simulink library "XtremeDSPKit"  (Simulink 7.1)
libraries: xbsIndex_r4 x66, dspindex x2, dspmtrx3 x2
settings Model: Creator=shirazi  LastModifiedBy=sysgengroup

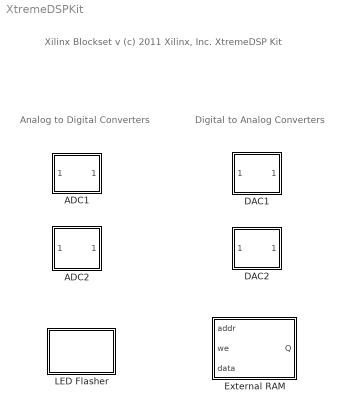
== system XtremeDSPKit ==
  note: Analog to Digital Converters
  note: Digital to Analog Converters
  note: Xilinx Blockset v
      | (c) 2011 Xilinx, Inc.
      |
      | XtremeDSP Kit
  ADC1 : Subsystem  mask(XtremeDSP Kit ADC1){period=1}
      mask prompts: period "Sample Period"
      mask help: Analog to Digital Converter #1
      mask init:
      | i = imread('xtreme.jpg');
      mask Help: eval('');xlDoc('-book','sysgen','-topic','XtremeDSP_Analog_to_Digital_Converter');
      mask Display: image(i)
  ADC2 : Subsystem  mask(XtremeDSP Kit  ADC2){period=1}
      mask prompts: period "Sample Period"
      mask help: Analog to Digital Converter #2
      mask init:
      | i = imread('xtreme.jpg');
      mask Help: eval('');xlDoc('-book','sysgen','-topic','XtremeDSP_Analog_to_Digital_Converter');
      mask Display: image(i)
  DAC1 : Subsystem  mask(XtremeDSP Kit DAC1){period=1}
      mask prompts: period "Sample Period"
      mask help: Digital to Analog Converter #1
      mask init:
      | i = imread('xtreme.jpg');
      mask Help: eval('');xlDoc('-book','sysgen','-topic','XtremeDSP_Digital_to_Analog_Converter');
      mask Display: image(i)
  DAC2 : Subsystem  mask(XtremeDSP Kit DAC2){period=1}
      mask prompts: period "Sample Period"
      mask help: Digital to Analog Converter #2
      mask init:
      | i = imread('xtreme.jpg');
      mask Help: eval('');xlDoc('-book','sysgen','-topic','XtremeDSP_Digital_to_Analog_Converter');
      mask Display: image(i)
  External RAM : Subsystem  mask(XtremeDSP Kit External Memory){zbt_data_read_arith_type=Unsigned, zbt_data_width=16, zbt_data_bin_pt=0}
      mask prompts: zbt_data_read_arith_type "Output Data Type"; zbt_data_width "Data Width"; zbt_data_bin_pt "Data Binary Point (from 0 to 16)"
      mask help: 256K x 16 External Memory
      mask init:
      | i = imread('xtreme.jpg');
      mask Help: eval('');xlDoc('-book','sysgen','-topic','XtremeDSP_External_RAM');
      mask StyleString: popup(Unsigned|Signed  (2's comp)),edit,edit
      mask Display:
      | image(i);
      | port_label ('input', 1, 'addr');
      | port_label ('input', 2, 'we');
      | port_label ('input', 3, 'data');
  LED Flasher : Subsystem  mask(LED Flasher){}
      mask help: This block will cause LEDs on the BenAdda to cycle through red, green, and yellow colors.
      mask init:
      | i = imread('LEDs.jpg');
      mask Help: eval('');xlDoc('-book','sysgen','-topic','XtremeDSP_LED_Flasher');
      mask Display: image(i)

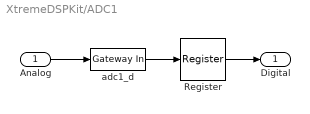
== system XtremeDSPKit/ADC1 ==
  Analog : Inport  OutDataType=sfix(16)  OutScaling=2^0
  Register : xbsIndex_r4/Register  init=0  rst=off  en=off  dbl_ovrd=off  block_type=register
      settings: xl_area=[0, 0, 0, 0, 0, 0, 0]  block_version=VER_STRING_GOES_HERE
  adc1_d : xbsIndex_r4/Gateway In  arith_type="Signed  (2's comp)"  n_bits=14  bin_pt=13  quantization="Round  (unbiased: +/- Inf)"  overflow=Saturate  period=period  dbl_ovrd=off  timing_constraint=None  locs_specified=off  LOCs={'w15', 'w14', 'w13', 'y15', 'y14', 'aa13', 'aa15', 'ab15', 'ac15', 'ad15', 'ac19', 'ac22', 'ad19', 'af20'}  block_type=gatewayin
      settings: infoedit="Gateway in block.  Converts inputs of type Simulink integer, double and fixed point to  Xilinx fixed point type.<P><P>Hardware notes:  In hardware these blocks become top level input ports."  xl_area=[0, 0, 0, 0, 0, 0, 0]  sginterface={'Nallatech'=>{'xdspkit'=>{'non_memory_mapped_port'=>'adc1_d'}},'Xilinx'=>{'jtaghwcosim'=>{'non_memory_mapped_port'=>'adc1_d'},'xdspkit'=>{'non_memory_mapped_port'=>'adc1_d'}}}  block_version=VER_STRING_GOES_HERE
  Digital : Outport  OutDataType=sfix(16)  OutScaling=2^0
  wires:
  Analog/1 -> adc1_d/1
  Register/1 -> Digital/1
  adc1_d/1 -> Register/1

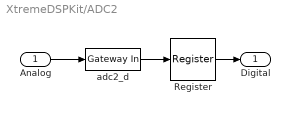
== system XtremeDSPKit/ADC2 ==
  Analog : Inport  OutDataType=sfix(16)  OutScaling=2^0
  Register : xbsIndex_r4/Register  init=0  rst=off  en=off  dbl_ovrd=off  block_type=register
      settings: xl_area=[0, 0, 0, 0, 0, 0, 0]  block_version=VER_STRING_GOES_HERE
  adc2_d : xbsIndex_r4/Gateway In  arith_type="Signed  (2's comp)"  n_bits=14  bin_pt=13  quantization="Round  (unbiased: +/- Inf)"  overflow=Saturate  period=period  dbl_ovrd=off  timing_constraint=None  locs_specified=off  LOCs={'w12', 'y10', 'y8', 'aa8', 'aa7', 'ab8', 'ab7', 'ab6', 'ac7', 'ac6', 'ac5', 'ad7', 'ad6', 'ad12'}  block_type=gatewayin
      settings: infoedit="Gateway in block.  Converts inputs of type Simulink integer, double and fixed point to  Xilinx fixed point type.<P><P>Hardware notes:  In hardware these blocks become top level input ports."  xl_area=[0, 0, 0, 0, 0, 0, 0]  sginterface={'Nallatech'=>{'xdspkit'=>{'non_memory_mapped_port'=>'adc2_d'}},'Xilinx'=>{'jtaghwcosim'=>{'non_memory_mapped_port'=>'adc2_d'},'xdspkit'=>{'non_memory_mapped_port'=>'adc2_d'}}}  block_version=VER_STRING_GOES_HERE
  Digital : Outport  OutDataType=sfix(16)  OutScaling=2^0
  wires:
  Analog/1 -> adc2_d/1
  Register/1 -> Digital/1
  adc2_d/1 -> Register/1

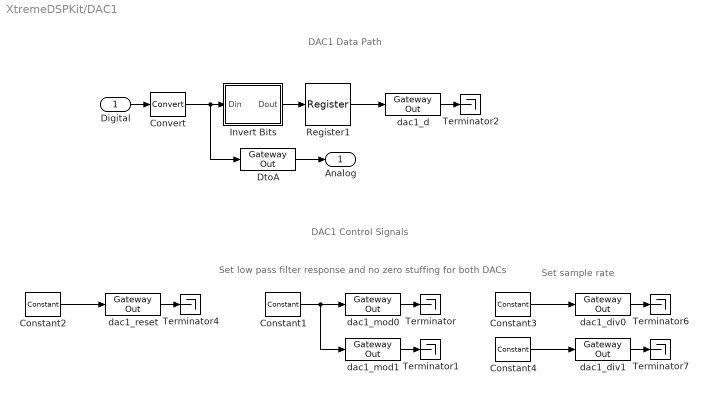
== system XtremeDSPKit/DAC1 ==
  note: DAC1 Data Path
  note: DAC1 Control Signals
  note: Set low pass filter response and
      | no zero stuffing for both DACs
  note: Set sample rate
  Digital : Inport  OutDataType=sfix(16)  OutScaling=2^0
  Constant1 : xbsIndex_r4/Constant  arith_type=Unsigned  const=0  n_bits=1  bin_pt=0  explicit_period=on  period=period  equ=P=C  opselect=C  inp2=PCIN>>17  opr=+  inp1=P  carry=CIN  dbl_ovrd=off  block_type=constant
      settings: block_version=VER_STRING_GOES_HERE
  Constant2 : xbsIndex_r4/Constant  arith_type=Unsigned  const=0  n_bits=1  bin_pt=0  explicit_period=on  period=period  equ=P=C  opselect=C  inp2=PCIN>>17  opr=+  inp1=P  carry=CIN  dbl_ovrd=off  block_type=constant
      settings: block_version=VER_STRING_GOES_HERE
  Constant3 : xbsIndex_r4/Constant  arith_type=Unsigned  const=1  n_bits=1  bin_pt=0  explicit_period=on  period=period  equ=P=C  opselect=C  inp2=PCIN>>17  opr=+  inp1=P  carry=CIN  dbl_ovrd=off  block_type=constant
      settings: block_version=VER_STRING_GOES_HERE
  Constant4 : xbsIndex_r4/Constant  arith_type=Unsigned  const=0  n_bits=1  bin_pt=0  explicit_period=on  period=period  equ=P=C  opselect=C  inp2=PCIN>>17  opr=+  inp1=P  carry=CIN  dbl_ovrd=off  block_type=constant
      settings: block_version=VER_STRING_GOES_HERE
  Convert : xbsIndex_r4/Convert  arith_type="Signed  (2's comp)"  n_bits=14  bin_pt=13  quantization=Truncate  overflow=Wrap  latency=0  dbl_ovrd=off  pipeline=off  block_type=convert
      settings: infoedit=The input is presented at the output after quantization and overflow effects.<P><P>Hardware notes: Additional hardware is used when rounding or saturation is selected and output width is less than the input width.  xl_area=[0, 0, 0, 0, 0, 0, 0]  block_version=VER_STRING_GOES_HERE
  DtoA : xbsIndex_r4/Gateway Out  hdl_port=off  timing_constraint=None  locs_specified=off  LOCs={}  block_type=gatewayout
      settings: infoedit="Gateway out block.  Converts Xilinx fixed point inputs into ouputs of type Simulink integer, double, or fixed point.<P><P>Hardware notes:  In hardware these blocks become top level output ports or are discarded, depending on how they are configured."  xl_area=[0, 0, 0, 0, 0, 0, 0]  block_version=VER_STRING_GOES_HERE
  Invert Bits : Subsystem
  Register1 : xbsIndex_r4/Register  init=0  rst=off  en=off  dbl_ovrd=off  block_type=register
      settings: xl_area=[0, 0, 0, 0, 0, 0, 0]  block_version=VER_STRING_GOES_HERE
  Terminator{,1..2,4,6..7} (6 alike) : Terminator
  dac1_d : xbsIndex_r4/Gateway Out  hdl_port=on  timing_constraint=None  locs_specified=off  LOCs={'p19', 'p20', 'p21', 'p22', 'p23', 'r19', 'r23', 'r24', 't19', 'u21', 'u22', 'u23', 'u24', 'v24'}  block_type=gatewayout
      settings: infoedit="Gateway out block.  Converts Xilinx fixed point inputs into ouputs of type Simulink integer, double, or fixed point.<P><P>Hardware notes:  In hardware these blocks become top level output ports or are discarded, depending on how they are configured."  xl_area=[0, 0, 0, 0, 0, 0, 0]  sginterface={'Nallatech'=>{'xdspkit'=>{'non_memory_mapped_port'=>'dac1_d'}},'Xilinx'=>{'jtaghwcosim'=>{'non_memory_mapped_port'=>'dac1_d'},'xdspkit'=>{'non_memory_mapped_port'=>'dac1_d'}}}  block_version=VER_STRING_GOES_HERE
  dac1_div0 : xbsIndex_r4/Gateway Out  hdl_port=on  timing_constraint=None  locs_specified=off  LOCs={'t20'}  block_type=gatewayout
      settings: infoedit="Gateway out block.  Converts Xilinx fixed point inputs into ouputs of type Simulink integer, double, or fixed point.<P><P>Hardware notes:  In hardware these blocks become top level output ports or are discarded, depending on how they are configured."  xl_area=[0, 0, 0, 0, 0, 0, 0]  sginterface={'Nallatech'=>{'xdspkit'=>{'non_memory_mapped_port'=>'dac1_div0'}},'Xilinx'=>{'jtaghwcosim'=>{'non_memory_mapped_port'=>'dac1_div0'},'xdspkit'=>{'non_memory_mapped_port'=>'dac1_div0'}}}  block_version=VER_STRING_GOES_HERE
  dac1_div1 : xbsIndex_r4/Gateway Out  hdl_port=on  timing_constraint=None  locs_specified=off  LOCs={'t24'}  block_type=gatewayout
      settings: infoedit="Gateway out block.  Converts Xilinx fixed point inputs into ouputs of type Simulink integer, double, or fixed point.<P><P>Hardware notes:  In hardware these blocks become top level output ports or are discarded, depending on how they are configured."  xl_area=[0, 0, 0, 0, 0, 0, 0]  sginterface={'Nallatech'=>{'xdspkit'=>{'non_memory_mapped_port'=>'dac1_div1'}},'Xilinx'=>{'jtaghwcosim'=>{'non_memory_mapped_port'=>'dac1_div1'},'xdspkit'=>{'non_memory_mapped_port'=>'dac1_div1'}}}  block_version=VER_STRING_GOES_HERE
  dac1_mod0 : xbsIndex_r4/Gateway Out  hdl_port=on  timing_constraint=None  locs_specified=off  LOCs={'r21'}  block_type=gatewayout
      settings: infoedit="Gateway out block.  Converts Xilinx fixed point inputs into ouputs of type Simulink integer, double, or fixed point.<P><P>Hardware notes:  In hardware these blocks become top level output ports or are discarded, depending on how they are configured."  xl_area=[0, 0, 0, 0, 0, 0, 0]  sginterface={'Nallatech'=>{'xdspkit'=>{'non_memory_mapped_port'=>'dac1_mod0'}},'Xilinx'=>{'jtaghwcosim'=>{'non_memory_mapped_port'=>'dac1_mod0'},'xdspkit'=>{'non_memory_mapped_port'=>'dac1_mod0'}}}  block_version=VER_STRING_GOES_HERE
  dac1_mod1 : xbsIndex_r4/Gateway Out  hdl_port=on  timing_constraint=None  locs_specified=off  LOCs={'r22'}  block_type=gatewayout
      settings: infoedit="Gateway out block.  Converts Xilinx fixed point inputs into ouputs of type Simulink integer, double, or fixed point.<P><P>Hardware notes:  In hardware these blocks become top level output ports or are discarded, depending on how they are configured."  xl_area=[0, 0, 0, 0, 0, 0, 0]  sginterface={'Nallatech'=>{'xdspkit'=>{'non_memory_mapped_port'=>'dac1_mod1'}},'Xilinx'=>{'jtaghwcosim'=>{'non_memory_mapped_port'=>'dac1_mod1'},'xdspkit'=>{'non_memory_mapped_port'=>'dac1_mod1'}}}  block_version=VER_STRING_GOES_HERE
  dac1_reset : xbsIndex_r4/Gateway Out  hdl_port=on  timing_constraint=None  locs_specified=off  LOCs={'v23'}  block_type=gatewayout
      settings: infoedit="Gateway out block.  Converts Xilinx fixed point inputs into ouputs of type Simulink integer, double, or fixed point.<P><P>Hardware notes:  In hardware these blocks become top level output ports or are discarded, depending on how they are configured."  xl_area=[0, 0, 0, 0, 0, 0, 0]  sginterface={'Nallatech'=>{'xdspkit'=>{'non_memory_mapped_port'=>'dac1_reset'}},'Xilinx'=>{'jtaghwcosim'=>{'non_memory_mapped_port'=>'dac1_reset'},'xdspkit'=>{'non_memory_mapped_port'=>'dac1_reset'}}}  block_version=VER_STRING_GOES_HERE
  Analog : Outport  OutDataType=sfix(16)  OutScaling=2^0
  wires:
  DtoA/1 -> Analog/1
  dac1_d/1 -> Terminator2/1
  Constant4/1 -> dac1_div1/1
  dac1_div1/1 -> Terminator7/1
  dac1_div0/1 -> Terminator6/1
  Constant3/1 -> dac1_div0/1
  dac1_reset/1 -> Terminator4/1
  Constant2/1 -> dac1_reset/1
  dac1_mod1/1 -> Terminator1/1
  dac1_mod0/1 -> Terminator/1
  Constant1/1 -> dac1_mod1/1, dac1_mod0/1
  Digital/1 -> Convert/1
  Register1/1 -> dac1_d/1
  Invert Bits/1(Dout) -> Register1/1
  Convert/1 -> DtoA/1, Invert Bits/1(Din)

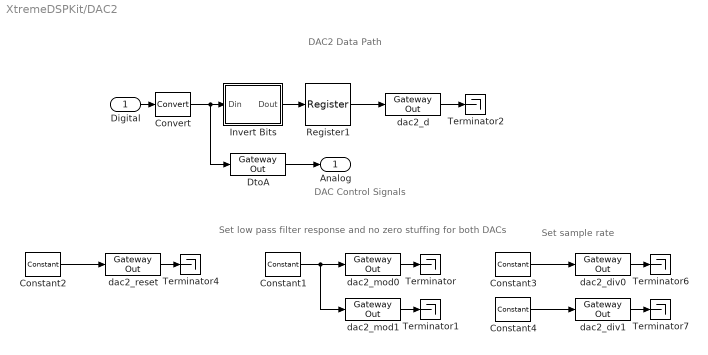
== system XtremeDSPKit/DAC2 ==
  note: Set sample rate
  note: Set low pass filter response and
      | no zero stuffing for both DACs
  note: DAC Control Signals
  note: DAC2 Data Path
  Digital : Inport  OutDataType=sfix(16)  OutScaling=2^0
  Constant1 : xbsIndex_r4/Constant  arith_type=Unsigned  const=0  n_bits=1  bin_pt=0  explicit_period=on  period=period  equ=P=C  opselect=C  inp2=PCIN>>17  opr=+  inp1=P  carry=CIN  dbl_ovrd=off  block_type=constant
      settings: block_version=VER_STRING_GOES_HERE
  Constant2 : xbsIndex_r4/Constant  arith_type=Unsigned  const=0  n_bits=1  bin_pt=0  explicit_period=on  period=period  equ=P=C  opselect=C  inp2=PCIN>>17  opr=+  inp1=P  carry=CIN  dbl_ovrd=off  block_type=constant
      settings: block_version=VER_STRING_GOES_HERE
  Constant3 : xbsIndex_r4/Constant  arith_type=Unsigned  const=1  n_bits=1  bin_pt=0  explicit_period=on  period=period  equ=P=C  opselect=C  inp2=PCIN>>17  opr=+  inp1=P  carry=CIN  dbl_ovrd=off  block_type=constant
      settings: block_version=VER_STRING_GOES_HERE
  Constant4 : xbsIndex_r4/Constant  arith_type=Unsigned  const=0  n_bits=1  bin_pt=0  explicit_period=on  period=period  equ=P=C  opselect=C  inp2=PCIN>>17  opr=+  inp1=P  carry=CIN  dbl_ovrd=off  block_type=constant
      settings: block_version=VER_STRING_GOES_HERE
  Convert : xbsIndex_r4/Convert  arith_type="Signed  (2's comp)"  n_bits=14  bin_pt=13  quantization=Truncate  overflow=Wrap  latency=0  dbl_ovrd=off  pipeline=off  block_type=convert
      settings: infoedit=The input is presented at the output after quantization and overflow effects.<P><P>Hardware notes: Additional hardware is used when rounding or saturation is selected and output width is less than the input width.  xl_area=[0, 0, 0, 0, 0, 0, 0]  block_version=VER_STRING_GOES_HERE
  DtoA : xbsIndex_r4/Gateway Out  hdl_port=off  timing_constraint=None  locs_specified=off  LOCs={}  block_type=gatewayout
      settings: infoedit="Gateway out block.  Converts Xilinx fixed point inputs into ouputs of type Simulink integer, double, or fixed point.<P><P>Hardware notes:  In hardware these blocks become top level output ports or are discarded, depending on how they are configured."  xl_area=[0, 0, 0, 0, 0, 0, 0]  block_version=VER_STRING_GOES_HERE
  Invert Bits : Subsystem
  Register1 : xbsIndex_r4/Register  init=0  rst=off  en=off  dbl_ovrd=off  block_type=register
      settings: xl_area=[0, 0, 0, 0, 0, 0, 0]  block_version=VER_STRING_GOES_HERE
  Terminator{,1..2,4,6..7} (6 alike) : Terminator
  dac2_d : xbsIndex_r4/Gateway Out  hdl_port=on  timing_constraint=None  locs_specified=off  LOCs={'y19', 'y20', 'y22', 'aa19', 'aa20', 'aa22', 'aa23', 'aa24', 'ab19', 'ab20', 'ab23', 'ab24', 'ac21', 'ad21'}  block_type=gatewayout
      settings: infoedit="Gateway out block.  Converts Xilinx fixed point inputs into ouputs of type Simulink integer, double, or fixed point.<P><P>Hardware notes:  In hardware these blocks become top level output ports or are discarded, depending on how they are configured."  xl_area=[0, 0, 0, 0, 0, 0, 0]  sginterface={'Nallatech'=>{'xdspkit'=>{'non_memory_mapped_port'=>'dac2_d'}},'Xilinx'=>{'jtaghwcosim'=>{'non_memory_mapped_port'=>'dac2_d'},'xdspkit'=>{'non_memory_mapped_port'=>'dac2_d'}}}  block_version=VER_STRING_GOES_HERE
  dac2_div0 : xbsIndex_r4/Gateway Out  hdl_port=on  timing_constraint=None  locs_specified=off  LOCs={'ac17'}  block_type=gatewayout
      settings: infoedit="Gateway out block.  Converts Xilinx fixed point inputs into ouputs of type Simulink integer, double, or fixed point.<P><P>Hardware notes:  In hardware these blocks become top level output ports or are discarded, depending on how they are configured."  xl_area=[0, 0, 0, 0, 0, 0, 0]  sginterface={'Nallatech'=>{'xdspkit'=>{'non_memory_mapped_port'=>'dac2_div0'}},'Xilinx'=>{'jtaghwcosim'=>{'non_memory_mapped_port'=>'dac2_div0'},'xdspkit'=>{'non_memory_mapped_port'=>'dac2_div0'}}}  block_version=VER_STRING_GOES_HERE
  dac2_div1 : xbsIndex_r4/Gateway Out  hdl_port=on  timing_constraint=None  locs_specified=off  LOCs={'ad17'}  block_type=gatewayout
      settings: infoedit="Gateway out block.  Converts Xilinx fixed point inputs into ouputs of type Simulink integer, double, or fixed point.<P><P>Hardware notes:  In hardware these blocks become top level output ports or are discarded, depending on how they are configured."  xl_area=[0, 0, 0, 0, 0, 0, 0]  sginterface={'Nallatech'=>{'xdspkit'=>{'non_memory_mapped_port'=>'dac2_div1'}},'Xilinx'=>{'jtaghwcosim'=>{'non_memory_mapped_port'=>'dac2_div1'},'xdspkit'=>{'non_memory_mapped_port'=>'dac2_div1'}}}  block_version=VER_STRING_GOES_HERE
  dac2_mod0 : xbsIndex_r4/Gateway Out  hdl_port=on  timing_constraint=None  locs_specified=off  LOCs={'t22'}  block_type=gatewayout
      settings: infoedit="Gateway out block.  Converts Xilinx fixed point inputs into ouputs of type Simulink integer, double, or fixed point.<P><P>Hardware notes:  In hardware these blocks become top level output ports or are discarded, depending on how they are configured."  xl_area=[0, 0, 0, 0, 0, 0, 0]  sginterface={'Nallatech'=>{'xdspkit'=>{'non_memory_mapped_port'=>'dac2_mod0'}},'Xilinx'=>{'jtaghwcosim'=>{'non_memory_mapped_port'=>'dac2_mod0'},'xdspkit'=>{'non_memory_mapped_port'=>'dac2_mod0'}}}  block_version=VER_STRING_GOES_HERE
  dac2_mod1 : xbsIndex_r4/Gateway Out  hdl_port=on  timing_constraint=None  locs_specified=off  LOCs={'t21'}  block_type=gatewayout
      settings: infoedit="Gateway out block.  Converts Xilinx fixed point inputs into ouputs of type Simulink integer, double, or fixed point.<P><P>Hardware notes:  In hardware these blocks become top level output ports or are discarded, depending on how they are configured."  xl_area=[0, 0, 0, 0, 0, 0, 0]  sginterface={'Nallatech'=>{'xdspkit'=>{'non_memory_mapped_port'=>'dac2_mod1'}},'Xilinx'=>{'jtaghwcosim'=>{'non_memory_mapped_port'=>'dac2_mod1'},'xdspkit'=>{'non_memory_mapped_port'=>'dac2_mod1'}}}  block_version=VER_STRING_GOES_HERE
  dac2_reset : xbsIndex_r4/Gateway Out  hdl_port=on  timing_constraint=None  locs_specified=off  LOCs={'u20'}  block_type=gatewayout
      settings: infoedit="Gateway out block.  Converts Xilinx fixed point inputs into ouputs of type Simulink integer, double, or fixed point.<P><P>Hardware notes:  In hardware these blocks become top level output ports or are discarded, depending on how they are configured."  xl_area=[0, 0, 0, 0, 0, 0, 0]  sginterface={'Nallatech'=>{'xdspkit'=>{'non_memory_mapped_port'=>'dac2_reset'}},'Xilinx'=>{'jtaghwcosim'=>{'non_memory_mapped_port'=>'dac2_reset'},'xdspkit'=>{'non_memory_mapped_port'=>'dac2_reset'}}}  block_version=VER_STRING_GOES_HERE
  Analog : Outport  OutDataType=sfix(16)  OutScaling=2^0
  wires:
  DtoA/1 -> Analog/1
  dac2_d/1 -> Terminator2/1
  Invert Bits/1(Dout) -> Register1/1
  Register1/1 -> dac2_d/1
  Digital/1 -> Convert/1
  Constant1/1 -> dac2_mod0/1, dac2_mod1/1
  dac2_mod0/1 -> Terminator/1
  dac2_mod1/1 -> Terminator1/1
  Constant2/1 -> dac2_reset/1
  dac2_reset/1 -> Terminator4/1
  Constant3/1 -> dac2_div0/1
  dac2_div0/1 -> Terminator6/1
  dac2_div1/1 -> Terminator7/1
  Constant4/1 -> dac2_div1/1
  Convert/1 -> DtoA/1, Invert Bits/1(Din)

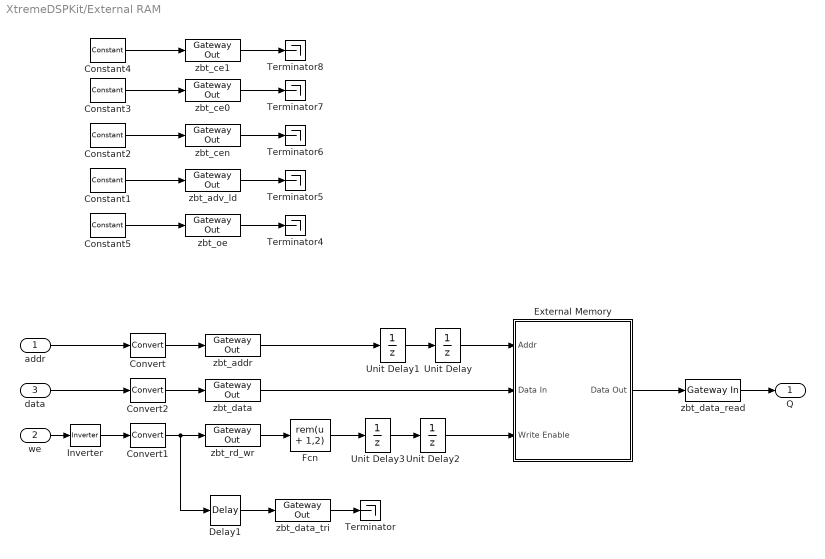
== system XtremeDSPKit/External RAM ==
  addr : Inport  OutDataType=sfix(16)  OutScaling=2^0
  we : Inport  Port=2  OutDataType=sfix(16)  OutScaling=2^0
  data : Inport  Port=3  OutDataType=sfix(16)  OutScaling=2^0
  Constant{1..5} (5 alike) : xbsIndex_r4/Constant  arith_type=Unsigned  const=0  n_bits=1  bin_pt=0  explicit_period=on  period=1  equ=P=C  opselect=C  inp2=PCIN>>17  opr=+  inp1=P  carry=CIN  dbl_ovrd=off  block_type=constant
      settings: block_version=VER_STRING_GOES_HERE
  Convert : xbsIndex_r4/Convert  arith_type=Unsigned  n_bits=18  bin_pt=0  quantization=Truncate  overflow=Wrap  latency=0  dbl_ovrd=off  pipeline=off  block_type=convert
      settings: infoedit=The input is presented at the output after quantization and overflow effects.<P><P>Hardware notes: Additional hardware is used when rounding or saturation is selected and output width is less than the input width.  xl_area=[0, 0, 0, 0, 0, 0, 0]  block_version=VER_STRING_GOES_HERE
  Convert1 : xbsIndex_r4/Convert  arith_type=Boolean  n_bits=1  bin_pt=0  quantization=Truncate  overflow=Wrap  latency=0  dbl_ovrd=off  pipeline=off  block_type=convert
      settings: infoedit=The input is presented at the output after quantization and overflow effects.<P><P>Hardware notes: Additional hardware is used when rounding or saturation is selected and output width is less than the input width.  xl_area=[0, 0, 0, 0, 0, 0, 0]  block_version=VER_STRING_GOES_HERE
  Convert2 : xbsIndex_r4/Convert  arith_type="Signed  (2's comp)"  n_bits=zbt_data_width  bin_pt=zbt_data_bin_pt  quantization=Truncate  overflow=Wrap  latency=0  dbl_ovrd=off  pipeline=off  block_type=convert
      settings: infoedit=The input is presented at the output after quantization and overflow effects.<P><P>Hardware notes: Additional hardware is used when rounding or saturation is selected and output width is less than the input width.  xl_area=[0, 0, 0, 0, 0, 0, 0]  block_version=VER_STRING_GOES_HERE
  Delay1 : xbsIndex_r4/Delay  en=off  latency=2  dbl_ovrd=off  reg_retiming=off  block_type=delay
      settings: infoedit="Delay line having  configurable length.<P><P>Hardware notes: A delay line is a chain, each link of which is an SRL16 followed by a flip-flop. If register retiming is enabled, the delay line is a chain of flip-flops."  xl_area=[0, 0, 0, 0, 0, 0, 0]  block_version=VER_STRING_GOES_HERE
  External Memory : Subsystem  mask{depth=4096, init_vec=0*(0:4095)}
      mask prompts: depth "Memory Depth"; init_vec "Initial Value"
  Fcn : Fcn  Expr=rem(u + 1,2)
  Inverter : xbsIndex_r4/Inverter  en=off  latency=0  dbl_ovrd=off  block_type=inv
      settings: xl_area=[0, 0, 0, 0, 0, 0, 0]  block_version=VER_STRING_GOES_HERE
  Terminator{,4..8} (6 alike) : Terminator
  Unit Delay{,1..3} (4 alike) : UnitDelay
  zbt_addr : xbsIndex_r4/Gateway Out  hdl_port=on  timing_constraint=None  locs_specified=off  LOCs={'A5','B9','A9','C1','A3','G6','E9','A6','A7','A8','B8','B1','B3','D9','B5','B4','B6','C2'}  block_type=gatewayout
      settings: infoedit="Gateway out block.  Converts Xilinx fixed point inputs into ouputs of type Simulink integer, double, or fixed point.<P><P>Hardware notes:  In hardware these blocks become top level output ports or are discarded, depending on how they are configured."  xl_area=[0, 0, 0, 0, 0, 0, 0]  sginterface={'Nallatech'=>{'xdspkit'=>{'non_memory_mapped_port'=>'zbt_addr'}},'Xilinx'=>{'jtaghwcosim'=>{'non_memory_mapped_port'=>'zbt_addr'},'xdspkit'=>{'non_memory_mapped_port'=>'zbt_addr'}}}  block_version=VER_STRING_GOES_HERE
  zbt_adv_ld : xbsIndex_r4/Gateway Out  hdl_port=on  timing_constraint=None  locs_specified=off  LOCs={'B15'}  block_type=gatewayout
      settings: infoedit="Gateway out block.  Converts Xilinx fixed point inputs into ouputs of type Simulink integer, double, or fixed point.<P><P>Hardware notes:  In hardware these blocks become top level output ports or are discarded, depending on how they are configured."  xl_area=[0, 0, 0, 0, 0, 0, 0]  sginterface={'Nallatech'=>{'xdspkit'=>{'non_memory_mapped_port'=>'zbt_adv_ld'}},'Xilinx'=>{'jtaghwcosim'=>{'non_memory_mapped_port'=>'zbt_adv_ld'},'xdspkit'=>{'non_memory_mapped_port'=>'zbt_adv_ld'}}}  block_version=VER_STRING_GOES_HERE
  zbt_ce0 : xbsIndex_r4/Gateway Out  hdl_port=on  timing_constraint=None  locs_specified=off  LOCs={'A18'}  block_type=gatewayout
      settings: infoedit="Gateway out block.  Converts Xilinx fixed point inputs into ouputs of type Simulink integer, double, or fixed point.<P><P>Hardware notes:  In hardware these blocks become top level output ports or are discarded, depending on how they are configured."  xl_area=[0, 0, 0, 0, 0, 0, 0]  sginterface={'Nallatech'=>{'xdspkit'=>{'non_memory_mapped_port'=>'zbt_ce0'}},'Xilinx'=>{'jtaghwcosim'=>{'non_memory_mapped_port'=>'zbt_ce0'},'xdspkit'=>{'non_memory_mapped_port'=>'zbt_ce0'}}}  block_version=VER_STRING_GOES_HERE
  zbt_ce1 : xbsIndex_r4/Gateway Out  hdl_port=on  timing_constraint=None  locs_specified=off  LOCs={'A19'}  block_type=gatewayout
      settings: infoedit="Gateway out block.  Converts Xilinx fixed point inputs into ouputs of type Simulink integer, double, or fixed point.<P><P>Hardware notes:  In hardware these blocks become top level output ports or are discarded, depending on how they are configured."  xl_area=[0, 0, 0, 0, 0, 0, 0]  sginterface={'Nallatech'=>{'xdspkit'=>{'non_memory_mapped_port'=>'zbt_ce1'}},'Xilinx'=>{'jtaghwcosim'=>{'non_memory_mapped_port'=>'zbt_ce1'},'xdspkit'=>{'non_memory_mapped_port'=>'zbt_ce1'}}}  block_version=VER_STRING_GOES_HERE
  zbt_cen : xbsIndex_r4/Gateway Out  hdl_port=on  timing_constraint=None  locs_specified=off  LOCs={'C15'}  block_type=gatewayout
      settings: infoedit="Gateway out block.  Converts Xilinx fixed point inputs into ouputs of type Simulink integer, double, or fixed point.<P><P>Hardware notes:  In hardware these blocks become top level output ports or are discarded, depending on how they are configured."  xl_area=[0, 0, 0, 0, 0, 0, 0]  sginterface={'Nallatech'=>{'xdspkit'=>{'non_memory_mapped_port'=>'zbt_cen'}},'Xilinx'=>{'jtaghwcosim'=>{'non_memory_mapped_port'=>'zbt_cen'},'xdspkit'=>{'non_memory_mapped_port'=>'zbt_cen'}}}  block_version=VER_STRING_GOES_HERE
  zbt_data : xbsIndex_r4/Gateway Out  hdl_port=on  timing_constraint=None  locs_specified=off  LOCs={'B21','B22','A22','B23','B19','C19','A20','A21','A23','B24','A24','A25','E18','D18','C18','B18'}  block_type=gatewayout
      settings: infoedit="Gateway out block.  Converts Xilinx fixed point inputs into ouputs of type Simulink integer, double, or fixed point.<P><P>Hardware notes:  In hardware these blocks become top level output ports or are discarded, depending on how they are configured."  xl_area=[0, 0, 0, 0, 0, 0, 0]  sginterface={'Nallatech'=>{'xdspkit'=>{'non_memory_mapped_port'=>'zbt_data'}},'Xilinx'=>{'jtaghwcosim'=>{'non_memory_mapped_port'=>'zbt_data'},'xdspkit'=>{'non_memory_mapped_port'=>'zbt_data'}}}  block_version=VER_STRING_GOES_HERE
  zbt_data_read : xbsIndex_r4/Gateway In  arith_type_sgadvanced=zbt_data_read_arith_type  arith_type=Unsigned  n_bits=zbt_data_width  bin_pt=zbt_data_bin_pt  quantization="Round  (unbiased: +/- Inf)"  overflow=Saturate  period=1  dbl_ovrd=off  timing_constraint=None  locs_specified=off  LOCs={}  block_type=gatewayin
      settings: infoedit="Gateway in block.  Converts inputs of type Simulink integer, double and fixed point to  Xilinx fixed point type.<P><P>Hardware notes:  In hardware these blocks become top level input ports."  xl_area=[0, 0, 0, 0, 0, 0, 0]  sginterface={'Nallatech'=>{'xdspkit'=>{'non_memory_mapped_port'=>'zbt_data_read'}},'Xilinx'=>{'jtaghwcosim'=>{'non_memory_mapped_port'=>'zbt_data_read'},'xdspkit'=>{'non_memory_mapped_port'=>'zbt_data_read'}}}  has_advanced_control=1  block_version=VER_STRING_GOES_HERE
  zbt_data_tri : xbsIndex_r4/Gateway Out  hdl_port=on  timing_constraint=None  locs_specified=off  LOCs={}  block_type=gatewayout
      settings: infoedit="Gateway out block.  Converts Xilinx fixed point inputs into ouputs of type Simulink integer, double, or fixed point.<P><P>Hardware notes:  In hardware these blocks become top level output ports or are discarded, depending on how they are configured."  xl_area=[0, 0, 0, 0, 0, 0, 0]  sginterface={'Nallatech'=>{'xdspkit'=>{'non_memory_mapped_port'=>'zbt_data_tri'}},'Xilinx'=>{'jtaghwcosim'=>{'non_memory_mapped_port'=>'zbt_data_tri'},'xdspkit'=>{'non_memory_mapped_port'=>'zbt_data_tri'}}}  block_version=VER_STRING_GOES_HERE
  zbt_oe : xbsIndex_r4/Gateway Out  hdl_port=on  timing_constraint=None  locs_specified=off  LOCs={'A15'}  block_type=gatewayout
      settings: infoedit="Gateway out block.  Converts Xilinx fixed point inputs into ouputs of type Simulink integer, double, or fixed point.<P><P>Hardware notes:  In hardware these blocks become top level output ports or are discarded, depending on how they are configured."  xl_area=[0, 0, 0, 0, 0, 0, 0]  sginterface={'Nallatech'=>{'xdspkit'=>{'non_memory_mapped_port'=>'zbt_oe'}},'Xilinx'=>{'jtaghwcosim'=>{'non_memory_mapped_port'=>'zbt_oe'},'xdspkit'=>{'non_memory_mapped_port'=>'zbt_oe'}}}  block_version=VER_STRING_GOES_HERE
  zbt_rd_wr : xbsIndex_r4/Gateway Out  hdl_port=on  timing_constraint=None  locs_specified=off  LOCs={'A14'}  block_type=gatewayout
      settings: infoedit="Gateway out block.  Converts Xilinx fixed point inputs into ouputs of type Simulink integer, double, or fixed point.<P><P>Hardware notes:  In hardware these blocks become top level output ports or are discarded, depending on how they are configured."  xl_area=[0, 0, 0, 0, 0, 0, 0]  sginterface={'Nallatech'=>{'xdspkit'=>{'non_memory_mapped_port'=>'zbt_rd_wr'}},'Xilinx'=>{'jtaghwcosim'=>{'non_memory_mapped_port'=>'zbt_rd_wr'},'xdspkit'=>{'non_memory_mapped_port'=>'zbt_rd_wr'}}}  block_version=VER_STRING_GOES_HERE
  Q : Outport  OutDataType=sfix(16)  OutScaling=2^0
  wires:
  Convert2/1 -> zbt_data/1
  Convert1/1 -> Delay1/1, zbt_rd_wr/1
  Convert/1 -> zbt_addr/1
  External Memory/1(Data Out) -> zbt_data_read/1
  zbt_data/1 -> External Memory/2(Data In)
  Unit Delay2/1 -> External Memory/3(Write Enable)
  Unit Delay3/1 -> Unit Delay2/1
  zbt_addr/1 -> Unit Delay1/1
  Unit Delay1/1 -> Unit Delay/1
  Unit Delay/1 -> External Memory/1(Addr)
  we/1 -> Inverter/1
  addr/1 -> Convert/1
  Constant5/1 -> zbt_oe/1
  Constant4/1 -> zbt_ce1/1
  zbt_ce1/1 -> Terminator8/1
  Constant3/1 -> zbt_ce0/1
  zbt_ce0/1 -> Terminator7/1
  Constant2/1 -> zbt_cen/1
  zbt_cen/1 -> Terminator6/1
  Constant1/1 -> zbt_adv_ld/1
  zbt_adv_ld/1 -> Terminator5/1
  zbt_oe/1 -> Terminator4/1
  zbt_data_read/1 -> Q/1
  zbt_data_tri/1 -> Terminator/1
  Delay1/1 -> zbt_data_tri/1
  data/1 -> Convert2/1
  zbt_rd_wr/1 -> Fcn/1
  Fcn/1 -> Unit Delay3/1
  Inverter/1 -> Convert1/1

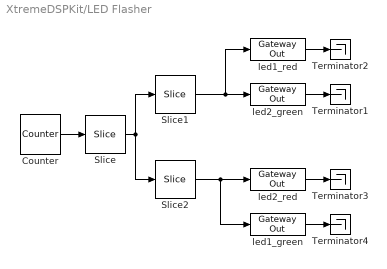
== system XtremeDSPKit/LED Flasher ==
  Counter : xbsIndex_r4/Counter  cnt_type=Free Running  cnt_to=Inf  operation=Up  start_count=0  cnt_by_val=1  arith_type="Signed  (2's comp)"  n_bits=27  bin_pt=0  load_pin=off  rst=off  en=off  explicit_period=off  period=1  dbl_ovrd=off  use_behavioral_HDL=off  use_rpm=off  block_type=counter
      settings: infoedit="Configurable up, down and up/down counter.<P><P>Hardware notes: Free running counters are the least expensive in hardware.  A count limited counter is implemented by combining a counter with a comparator."  xl_area=[0, 0, 0, 0, 0, 0, 0]  block_version=VER_STRING_GOES_HERE
  Slice : xbsIndex_r4/Slice  nbits=2  boolean_output=off  mode=Upper Bit Location + Width  bit1=0  base1=MSB of Input  bit0=0  base0=LSB of Input  dbl_ovrd=off  block_type=slice
      settings: infoedit="Extracts a given range of bits from each input sample and presents it at the output.  The output type is ordinarily unsigned with binary point at zero, but can be Boolean when the slice is one bit wide.<P><P>Hardware notes: In hardware this block costs nothing."  block_version=VER_STRING_GOES_HERE
  Slice1 : xbsIndex_r4/Slice  nbits=1  boolean_output=off  mode=Upper Bit Location + Width  bit1=0  base1=MSB of Input  bit0=0  base0=LSB of Input  dbl_ovrd=off  block_type=slice
      settings: infoedit="Extracts a given range of bits from each input sample and presents it at the output.  The output type is ordinarily unsigned with binary point at zero, but can be Boolean when the slice is one bit wide.<P><P>Hardware notes: In hardware this block costs nothing."  block_version=VER_STRING_GOES_HERE
  Slice2 : xbsIndex_r4/Slice  nbits=1  boolean_output=off  mode=Lower Bit Location + Width  bit1=0  base1=MSB of Input  bit0=0  base0=LSB of Input  dbl_ovrd=off  block_type=slice
      settings: infoedit="Extracts a given range of bits from each input sample and presents it at the output.  The output type is ordinarily unsigned with binary point at zero, but can be Boolean when the slice is one bit wide.<P><P>Hardware notes: In hardware this block costs nothing."  block_version=VER_STRING_GOES_HERE
  Terminator{1..4} (4 alike) : Terminator
  led1_green : xbsIndex_r4/Gateway Out  hdl_port=on  timing_constraint=None  locs_specified=off  LOCs={'y23'}  block_type=gatewayout
      settings: infoedit="Gateway out block.  Converts Xilinx fixed point inputs into ouputs of type Simulink integer, double, or fixed point.<P><P>Hardware notes:  In hardware these blocks become top level output ports or are discarded, depending on how they are configured."  xl_area=[0, 0, 0, 0, 0, 0, 0]  sginterface={'Nallatech'=>{'xdspkit'=>{'non_memory_mapped_port'=>'led1_green'}},'Xilinx'=>{'jtaghwcosim'=>{'non_memory_mapped_port'=>'led1_green'},'xdspkit'=>{'non_memory_mapped_port'=>'led1_green'}}}  block_version=VER_STRING_GOES_HERE
  led1_red : xbsIndex_r4/Gateway Out  hdl_port=on  timing_constraint=None  locs_specified=off  LOCs={'y24'}  block_type=gatewayout
      settings: infoedit="Gateway out block.  Converts Xilinx fixed point inputs into ouputs of type Simulink integer, double, or fixed point.<P><P>Hardware notes:  In hardware these blocks become top level output ports or are discarded, depending on how they are configured."  xl_area=[0, 0, 0, 0, 0, 0, 0]  sginterface={'Nallatech'=>{'xdspkit'=>{'non_memory_mapped_port'=>'led1_red'}},'Xilinx'=>{'jtaghwcosim'=>{'non_memory_mapped_port'=>'led1_red'},'xdspkit'=>{'non_memory_mapped_port'=>'led1_red'}}}  block_version=VER_STRING_GOES_HERE
  led2_green : xbsIndex_r4/Gateway Out  hdl_port=on  timing_constraint=None  locs_specified=off  LOCs={'y11'}  block_type=gatewayout
      settings: infoedit="Gateway out block.  Converts Xilinx fixed point inputs into ouputs of type Simulink integer, double, or fixed point.<P><P>Hardware notes:  In hardware these blocks become top level output ports or are discarded, depending on how they are configured."  xl_area=[0, 0, 0, 0, 0, 0, 0]  sginterface={'Nallatech'=>{'xdspkit'=>{'non_memory_mapped_port'=>'led2_green'}},'Xilinx'=>{'jtaghwcosim'=>{'non_memory_mapped_port'=>'led2_green'},'xdspkit'=>{'non_memory_mapped_port'=>'led2_green'}}}  block_version=VER_STRING_GOES_HERE
  led2_red : xbsIndex_r4/Gateway Out  hdl_port=on  timing_constraint=None  locs_specified=off  LOCs={'aa11'}  block_type=gatewayout
      settings: infoedit="Gateway out block.  Converts Xilinx fixed point inputs into ouputs of type Simulink integer, double, or fixed point.<P><P>Hardware notes:  In hardware these blocks become top level output ports or are discarded, depending on how they are configured."  xl_area=[0, 0, 0, 0, 0, 0, 0]  sginterface={'Nallatech'=>{'xdspkit'=>{'non_memory_mapped_port'=>'led2_red'}},'Xilinx'=>{'jtaghwcosim'=>{'non_memory_mapped_port'=>'led2_red'},'xdspkit'=>{'non_memory_mapped_port'=>'led2_red'}}}  block_version=VER_STRING_GOES_HERE
  wires:
  Slice/1 -> Slice2/1, Slice1/1
  Counter/1 -> Slice/1
  led1_green/1 -> Terminator4/1
  led2_red/1 -> Terminator3/1
  led2_green/1 -> Terminator1/1
  led1_red/1 -> Terminator2/1
  Slice2/1 -> led1_green/1, led2_red/1
  Slice1/1 -> led2_green/1, led1_red/1

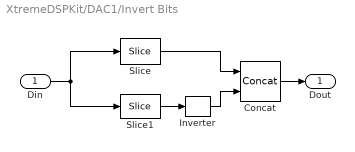
== system XtremeDSPKit/DAC1/Invert Bits ==
  Din : Inport  OutDataType=sfix(16)  OutScaling=2^0
  Concat : xbsIndex_r4/Concat  num_inputs=2  dbl_ovrd=off  block_type=concat
      settings: block_version=VER_STRING_GOES_HERE
  Inverter : xbsIndex_r4/Inverter  en=off  latency=0  dbl_ovrd=off  block_type=inv
      settings: xl_area=[0, 0, 0, 0, 0, 0, 0]  block_version=VER_STRING_GOES_HERE
  Slice : xbsIndex_r4/Slice  nbits=1  boolean_output=off  mode=Upper Bit Location + Width  bit1=0  base1=MSB of Input  bit0=0  base0=LSB of Input  dbl_ovrd=off  block_type=slice
      settings: infoedit="Extracts a given range of bits from each input sample and presents it at the output.  The output type is ordinarily unsigned with binary point at zero, but can be Boolean when the slice is one bit wide.<P><P>Hardware notes: In hardware this block costs nothing."  block_version=VER_STRING_GOES_HERE
  Slice1 : xbsIndex_r4/Slice  nbits=13  boolean_output=off  mode=Lower Bit Location + Width  bit1=0  base1=MSB of Input  bit0=0  base0=LSB of Input  dbl_ovrd=off  block_type=slice
      settings: infoedit="Extracts a given range of bits from each input sample and presents it at the output.  The output type is ordinarily unsigned with binary point at zero, but can be Boolean when the slice is one bit wide.<P><P>Hardware notes: In hardware this block costs nothing."  block_version=VER_STRING_GOES_HERE
  Dout : Outport  OutDataType=sfix(16)  OutScaling=2^0
  wires:
  Concat/1 -> Dout/1
  Slice1/1 -> Inverter/1
  Slice/1 -> Concat/1
  Din/1 -> Slice/1, Slice1/1
  Inverter/1 -> Concat/2

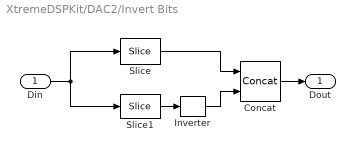
== system XtremeDSPKit/DAC2/Invert Bits ==
  Din : Inport  OutDataType=sfix(16)  OutScaling=2^0
  Concat : xbsIndex_r4/Concat  num_inputs=2  dbl_ovrd=off  block_type=concat
      settings: block_version=VER_STRING_GOES_HERE
  Inverter : xbsIndex_r4/Inverter  en=off  latency=0  dbl_ovrd=off  block_type=inv
      settings: xl_area=[0, 0, 0, 0, 0, 0, 0]  block_version=VER_STRING_GOES_HERE
  Slice : xbsIndex_r4/Slice  nbits=1  boolean_output=off  mode=Upper Bit Location + Width  bit1=0  base1=MSB of Input  bit0=0  base0=LSB of Input  dbl_ovrd=off  block_type=slice
      settings: infoedit="Extracts a given range of bits from each input sample and presents it at the output.  The output type is ordinarily unsigned with binary point at zero, but can be Boolean when the slice is one bit wide.<P><P>Hardware notes: In hardware this block costs nothing."  block_version=VER_STRING_GOES_HERE
  Slice1 : xbsIndex_r4/Slice  nbits=13  boolean_output=off  mode=Lower Bit Location + Width  bit1=0  base1=MSB of Input  bit0=0  base0=LSB of Input  dbl_ovrd=off  block_type=slice
      settings: infoedit="Extracts a given range of bits from each input sample and presents it at the output.  The output type is ordinarily unsigned with binary point at zero, but can be Boolean when the slice is one bit wide.<P><P>Hardware notes: In hardware this block costs nothing."  block_version=VER_STRING_GOES_HERE
  Dout : Outport  OutDataType=sfix(16)  OutScaling=2^0
  wires:
  Din/1 -> Slice1/1, Slice/1
  Slice/1 -> Concat/1
  Slice1/1 -> Inverter/1
  Concat/1 -> Dout/1
  Inverter/1 -> Concat/2

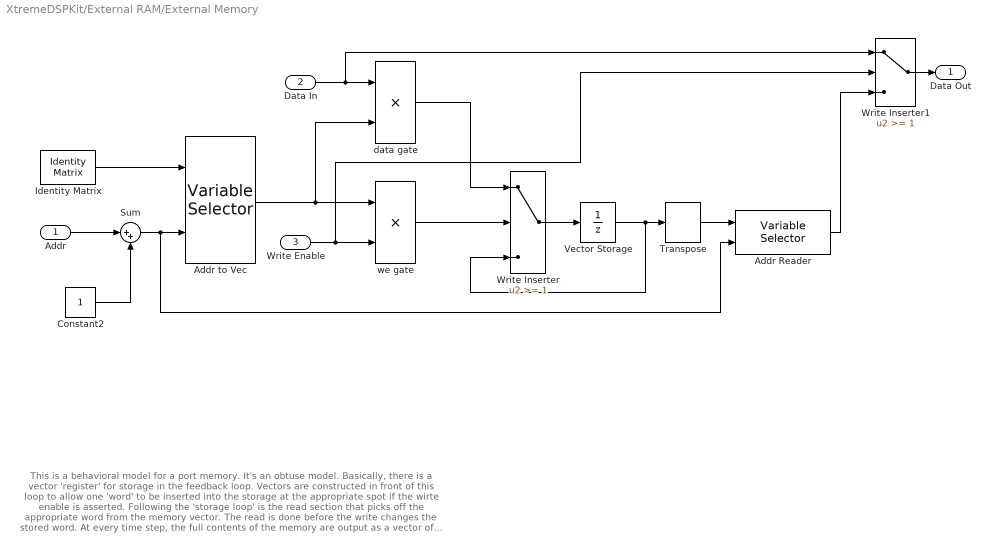
== system XtremeDSPKit/External RAM/External Memory ==
  note: This is a behavioral model for a port memory.
      | It's an obtuse model.  Basically, there is a vector 'register'
      | for storage in the feedback loop. Vectors are constructed
      | in front of this loop to allow one 'word' to be inserted into the
      | storage  at the appropriate spot if the wirte enable is
      | asserted.  Following the 'storage loop' is the read section
      | that picks off the appropriate word from the memory vector.
      |
      | The read is done before the write changes the stored word.
      |
      | At every time step, the full contents of the memory are output
      | as a  vector of doubles.  This is a very handy  feature  for
      | analysis and debugging.
  Addr : Inport  OutDataType=sfix(16)  OutScaling=2^0
  Data In : Inport  Port=2  OutDataType=sfix(16)  OutScaling=2^0
  Write Enable : Inport  Port=3  OutDataType=sfix(16)  OutScaling=2^0
  Addr Reader : dspindex/Variable Selector  NumInputs=1  rowsOrCols=Rows  IdxMode=Variable  Elements=[1 3]  ZerOneIdxMode=One-based  errmode=Generate Error  FillMode=on  FillValues=0
  Addr to Vec : dspindex/Variable Selector  NumInputs=1  rowsOrCols=Rows  IdxMode=Variable  Elements=[1 3]  ZerOneIdxMode=One-based  errmode=Clip Index  FillMode=on  FillValues=0
  Constant2 : Constant  OutDataType=sfix(16)  OutScaling=2^0
  Identity Matrix : dspmtrx3/Identity Matrix  Inherit=off  N=depth  Ts=1  dataType=double  isSigned=on  wordLen=16  udDataType=sfix(16)  fracBitsMode=Best precision  numFracBits=15
  Sum : Sum  Inputs=|++  OutDataType=sfix(16)  OutScaling=2^0  SaturateOnIntegerOverflow=on  InputSameDT=on  OutDataTypeStr=Inherit: Same as first input
  Transpose : dspmtrx3/Transpose  SystemSampleTime=-1  Hermitian=off  overflowFlag=on
  Vector Storage : UnitDelay  X0=init_vec
  Write Inserter : Switch  Threshold=1  SaturateOnIntegerOverflow=on  InputSameDT=on
  Write Inserter1 : Switch  Threshold=1  SaturateOnIntegerOverflow=on  InputSameDT=on
  data gate : Product  OutDataType=sfix(16)  OutScaling=2^0  SaturateOnIntegerOverflow=on  InputSameDT=on  OutDataTypeStr=Inherit: Same as first input
  we gate : Product  OutDataType=sfix(16)  OutScaling=2^0  SaturateOnIntegerOverflow=on  InputSameDT=on  OutDataTypeStr=Inherit: Same as first input
  Data Out : Outport  OutDataType=sfix(16)  OutScaling=2^0
  wires:
  Write Inserter1/1 -> Data Out/1
  Vector Storage/1 -> Transpose/1, Write Inserter/3
  Constant2/1 -> Sum/2
  Addr/1 -> Sum/1
  Sum/1 -> Addr Reader/2, Addr to Vec/2
  data gate/1 -> Write Inserter/1
  we gate/1 -> Write Inserter/2
  Data In/1 -> Write Inserter1/1, data gate/1
  Transpose/1 -> Addr Reader/1
  Write Enable/1 -> Write Inserter1/2, we gate/2
  Identity Matrix/1 -> Addr to Vec/1
  Addr to Vec/1 -> data gate/2, we gate/1
  Addr Reader/1 -> Write Inserter1/3
  Write Inserter/1 -> Vector Storage/1
